simulink model "tvcControlModel"  (R2017a)
settings: Solver=VariableStepAuto  StartTime=0.0  StopTime=inf  MaxStep=0.01  RelTol=1e-3
values from neighbouring files (symbols this model uses):
  A = 0.5    [script.m]
  Cd = 1.75    [script.m]
  g = 9.81    [script.m]
  m = 0.5    [script.m]
  r = 0.28    [script.m]
  rA = 1.229    [script.m]
  Th = 11.2    [script.m]
  time = 5    [script.m]
undefined symbols (not defined in the file or in its folder): sigbuilder_block
libraries: simulink_extras x7, simulink x7, shared3dof x1, aerolibanim x1
settings Model: Creator=Jafar Iqbal  LastModifiedBy=Jafar Iqbal
settings SolverCC: AlgebraicLoopSolver=LineSearch
settings HardwareCC: TargetBitPerPointer=64  TargetBitPerSizeT=64  TargetBitPerPtrDiffT=64  TargetLongLongMode=on  TargetIntDivRoundTo=Zero  TargetEndianess=LittleEndian  TargetWordSize=64  TargetHWDeviceType=MATLAB Host  ProdEqTarget=off
settings RTWCC: SystemTargetFile=rsim.tlc  TemplateMakefile=rsim_default_tmf  Description=Rapid Simulation Target  TargetLang=C++
settings RSimTargetCC: TargetLangStandard=C++03 (ISO)  GeneratePreprocessorConditionals=Use local settings

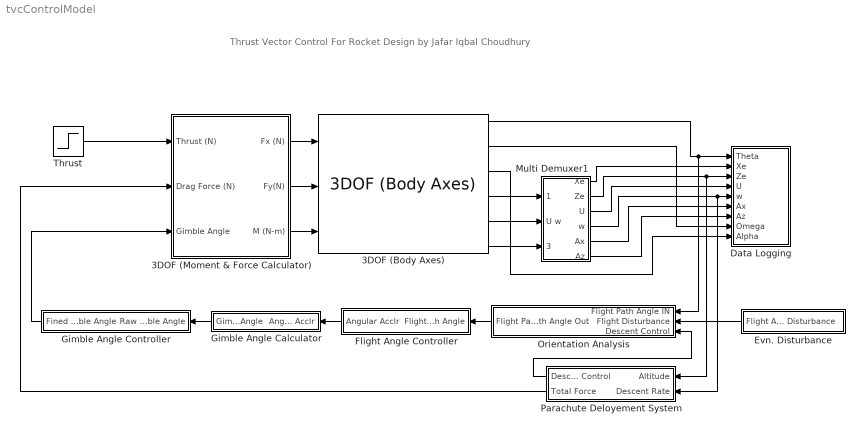
== system tvcControlModel ==
  note: Thrust Vector Control For Rocket
      | Design by Jafar Iqbal Choudhury
  3DOF (Body Axes) : shared3dof/3DOF (Body Axes)  units=Metric (MKS)  mtype=Fixed  v_ini=0  theta_ini=0  alpha_ini=0  q_ini=0  pos_ini=[0 0]  mass=m  mass_e=0.5  mass_f=3.0  Iyy=In  Iyy_e=0.5  Iyy_f=3.0  g_in=Internal  g=-9.81  vre_flag=on  abi_flag=off
  3DOF (Moment & Force Calculator) : Subsystem
  Data Logging : Subsystem
  Evn. Disturbance : Subsystem
  Flight Angle Controller : Subsystem
  Gimble Angle Calculator : Subsystem
  Gimble Angle Controller : Subsystem
  Multi Demuxer1 : Subsystem
  Orientation Analysis : Subsystem
  Parachute Deloyement System : Subsystem
  Thrust : Step  Time=time  Before=Th  After=0  SampleTime=0
  wires:
  3DOF (Moment & Force Calculator)/3(M (N-m)) -> 3DOF (Body Axes)/3
  3DOF (Moment & Force Calculator)/2(Fy(N)) -> 3DOF (Body Axes)/2
  3DOF (Moment & Force Calculator)/1(Fx (N)) -> 3DOF (Body Axes)/1
  Thrust/1 -> 3DOF (Moment & Force Calculator)/1(Thrust (N))
  3DOF (Body Axes)/4 -> Multi Demuxer1/1(Xe-Ze)
  3DOF (Body Axes)/5 -> Multi Demuxer1/2(U w)
  3DOF (Body Axes)/6 -> Multi Demuxer1/3(Ax - Az)
  Gimble Angle Controller/1(Fined Gimble Angle) -> 3DOF (Moment & Force Calculator)/3(Gimble Angle)
  Multi Demuxer1/2(Ze) -> Data Logging/3(Ze), Parachute Deloyement System/1(Altitude)
  3DOF (Body Axes)/1 -> Orientation Analysis/1(Flight Path Angle IN), Data Logging/1(Theta)
  Multi Demuxer1/1(Xe) -> Data Logging/2(Xe)
  Multi Demuxer1/3(U) -> Data Logging/4(U)
  Multi Demuxer1/5(Ax) -> Data Logging/6(Ax)
  Multi Demuxer1/6(Az) -> Data Logging/7(Az)
  3DOF (Body Axes)/2 -> Data Logging/8(Omega)
  3DOF (Body Axes)/3 -> Data Logging/9(Alpha)
  Multi Demuxer1/4(w) -> Parachute Deloyement System/2(Descent Rate), Data Logging/5(w)
  Evn. Disturbance/1(Flight Angle Disturbance) -> Orientation Analysis/2(Flight Disturbance)
  Gimble Angle Calculator/1(Gimble Angle) -> Gimble Angle Controller/1(Raw Gimble Angle)
  Flight Angle Controller/1(Angular Acclr) -> Gimble Angle Calculator/1(Angular Acclr)
  Orientation Analysis/1(Flight Path Angle Out) -> Flight Angle Controller/1(Flight Path Angle)
  Parachute Deloyement System/2(Total Force) -> 3DOF (Moment & Force Calculator)/2(Drag Force (N))
  Parachute Deloyement System/1(Descent Control) -> Orientation Analysis/3(Descent Control)

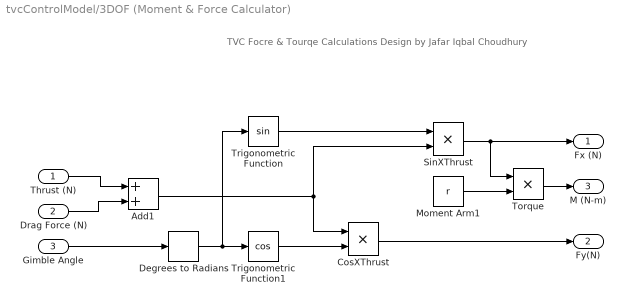
== system tvcControlModel/3DOF (Moment & Force Calculator) ==
  note: TVC Focre & Tourqe Calculations
      | Design by Jafar Iqbal Choudhury
  Thrust (N) : Inport
  Drag Force (N) : Inport  Port=2
  Gimble Angle : Inport  Port=3
  Add1 : Sum
  CosXThrust : Product
  Degrees to Radians : simulink_extras/Transformations/Degrees to Radians
  Moment Arm1 : Constant  Value=r
  SinXThrust : Product
  Torque : Product
  Trigonometric Function : Trigonometry
  Trigonometric Function1 : Trigonometry  Operator=cos
  Fx (N) : Outport
  Fy(N) : Outport  Port=2
  M (N-m) : Outport  Port=3
  wires:
  Degrees to Radians/1 -> Trigonometric Function/1, Trigonometric Function1/1
  SinXThrust/1 -> Torque/1, Fx (N)/1
  Trigonometric Function/1 -> SinXThrust/1
  Torque/1 -> M (N-m)/1
  Gimble Angle/1 -> Degrees to Radians/1
  Moment Arm1/1 -> Torque/2
  Trigonometric Function1/1 -> CosXThrust/2
  Thrust (N)/1 -> Add1/1
  Drag Force (N)/1 -> Add1/2
  Add1/1 -> SinXThrust/2, CosXThrust/1
  CosXThrust/1 -> Fy(N)/1

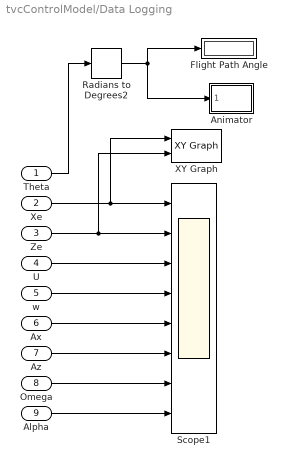
== system tvcControlModel/Data Logging ==
  Theta : Inport
  Xe : Inport  Port=2
  Ze : Inport  Port=3
  U : Inport  Port=4
  w : Inport  Port=5
  Ax : Inport  Port=6
  Az : Inport  Port=7
  Omega : Inport  Port=8
  Alpha : Inport  Port=9
  Animator : Subsystem
  Flight Path Angle : Display
  Radians to Degrees2 : simulink_extras/Transformations/Radians to Degrees
  Scope1 : Scope  NumInputPorts=8
  XY Graph : simulink/Sinks/XY Graph  xmin=-250  xmax=250  ymin=0  ymax=400  st=-1
  wires:
  Radians to Degrees2/1 -> Animator/1(FPA Input), Flight Path Angle/1
  Theta/1 -> Radians to Degrees2/1
  Ax/1 -> Scope1/5
  Az/1 -> Scope1/6
  Ze/1 -> XY Graph/2, Scope1/2
  Xe/1 -> XY Graph/1, Scope1/1
  Omega/1 -> Scope1/7
  Alpha/1 -> Scope1/8
  U/1 -> Scope1/3
  w/1 -> Scope1/4

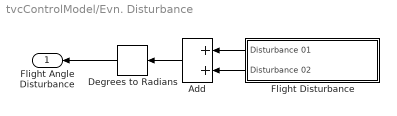
== system tvcControlModel/Evn. Disturbance ==
  Add : Sum
  Degrees to Radians : simulink_extras/Transformations/Degrees to Radians
  Flight Disturbance : Subsystem  Tag=STV Subsys  LoadFcn=sigbuilder_block('load');  StartFcn=sigbuilder_block('start');  StopFcn=sigbuilder_block('stop');  ClipboardFcn=sigbuilder_block('clipboard');  mask(Sigbuilder block){tuvar=[0:10]}
      mask help: Simulink:masks:SigbuilderBlock_MD
      mask init:
      | if ~strcmp(get_param(bdroot(gcbh),'SimulationStatus'),'stopped') tuvar = sigbuilder_block('maskInit'); end
      settings: CopyFcn=sigbuilder_block('copy');  DeleteFcn=sigbuilder_block('delete');  ModelCloseFcn=sigbuilder_block('modelClose');  PreSaveFcn=sigbuilder_block('preSave');  PauseFcn=sigbuilder_block('pause');  ContinueFcn=sigbuilder_block('continue');  NameChangeFcn=sigbuilder_block('namechange');  OpenFcn=sigbuilder_block('open',[309.75 207 550.5 483 ]);  CloseFcn=sigbuilder_block('close');
      mask Display: plot(0, 0, 100, 100,[2, 2, 32, 32, 2], [68, 8, 8, 68, 68],[32, 2], [38, 38], [32, 19, 2],[53, 60, 44], [32, 17, 17, 2],[16, 16, 31, 31]);txt = getActiveGroup(gcbh);text(2, 100, txt,'verticalAlignment', 'top');
  Flight Angle Disturbance : Outport
  wires:
  Degrees to Radians/1 -> Flight Angle Disturbance/1
  Flight Disturbance/1(Disturbance 01) -> Add/1
  Add/1 -> Degrees to Radians/1
  Flight Disturbance/2(Disturbance 02) -> Add/2

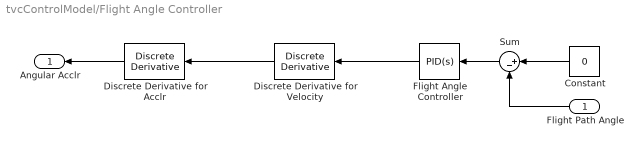
== system tvcControlModel/Flight Angle Controller ==
  Flight Path Angle : Inport
  Constant : Constant  Value=0
  Discrete Derivative for Acclr : simulink/Discrete/Discrete Derivative  gainval=1  ICPrevScaledInput=0.0  OutMin=[]  OutMax=[]  OutDataType=fixdt(1, 16)  OutScaling=2^-10  DoSatur=off
  Discrete Derivative for Velocity : simulink/Discrete/Discrete Derivative  gainval=0.5  ICPrevScaledInput=0.0  OutMin=[]  OutMax=[]  OutDataType=fixdt(1, 16)  OutScaling=2^-10  DoSatur=off
  Flight Angle Controller : simulink/Continuous/PID Controller  Controller=PID  TimeDomain=Continuous-time  SampleTime=-1  IntegratorMethod=Forward Euler  FilterMethod=Forward Euler  Form=Parallel  UseFilter=on  ControllerParametersSource=internal  P=0.179799982989109  I=4.81446374346561  D=-0.0354522581673334  N=5.07160875734514  InitialConditionSource=internal  InitialConditionForIntegrator=0  InitialConditionForFilter=0  ExternalReset=none  LimitOutput=off  UpperSaturationLimit=inf  LowerSaturationLimit=-inf  LinearizeAsGain=on  AntiWindupMode=none  Kb=1  TrackingMode=off  Kt=1  PParamMin=[]  PParamMax=[]  IParamMin=[]  IParamMax=[]  DParamMin=[]  DParamMax=[]  NParamMin=[]  NParamMax=[]  KbParamMin=[]  KbParamMax=[]  KtParamMin=[]  KtParamMax=[]  POutMin=[]  POutMax=[]  IOutMin=[]  IOutMax=[]  DOutMin=[]  DOutMax=[]  NOutMin=[]  NOutMax=[]  KbOutMin=[]  KbOutMax=[]  KtOutMin=[]  KtOutMax=[]  IntegratorOutMin=[]  IntegratorOutMax=[]  FilterOutMin=[]  FilterOutMax=[]  SumOutMin=[]  SumOutMax=[]  SumI1OutMin=[]  SumI1OutMax=[]  SumI2OutMin=[]  SumI2OutMax=[]  SumI3OutMin=[]  SumI3OutMax=[]  SumDOutMin=[]  SumDOutMax=[]  SaturationOutMin=[]  SaturationOutMax=[]  IntegratorContinuousStateAttributes=''  IntegratorStateMustResolveToSignalObject=off  IntegratorRTWStateStorageClass=Auto  FilterContinuousStateAttributes=''  FilterStateMustResolveToSignalObject=off  FilterRTWStateStorageClass=Auto  DifferentiatorICPrevScaledInput=0  DifferentiatorOutMin=[]  DifferentiatorOutMax=[]  InitialConditionSetting=State (most efficient)
  Sum : Sum  Inputs=|+-
  Angular Acclr : Outport
  wires:
  Discrete Derivative for Acclr/1 -> Angular Acclr/1
  Discrete Derivative for Velocity/1 -> Discrete Derivative for Acclr/1
  Flight Path Angle/1 -> Sum/2
  Sum/1 -> Flight Angle Controller/1
  Constant/1 -> Sum/1
  Flight Angle Controller/1 -> Discrete Derivative for Velocity/1

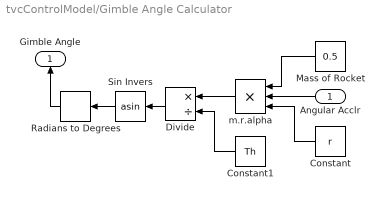
== system tvcControlModel/Gimble Angle Calculator ==
  Angular Acclr : Inport
  Constant : Constant  Value=r
  Constant1 : Constant  Value=Th
  Divide : Product  Inputs=*/
  Mass of Rocket : Constant  Value=0.5
  Radians to Degrees : simulink_extras/Transformations/Radians to Degrees
  Sin Invers : Trigonometry  Operator=asin
  m.r.alpha : Product  Inputs=3
  Gimble Angle : Outport
  wires:
  Constant/1 -> m.r.alpha/3
  Angular Acclr/1 -> m.r.alpha/2
  Divide/1 -> Sin Invers/1
  Sin Invers/1 -> Radians to Degrees/1
  Mass of Rocket/1 -> m.r.alpha/1
  m.r.alpha/1 -> Divide/1
  Radians to Degrees/1 -> Gimble Angle/1
  Constant1/1 -> Divide/2

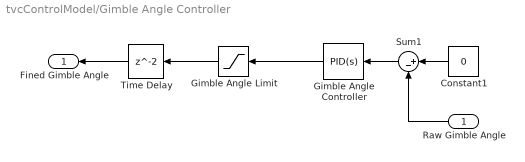
== system tvcControlModel/Gimble Angle Controller ==
  Raw Gimble Angle : Inport
  Constant1 : Constant  Value=0
  Gimble Angle Controller : simulink/Continuous/PID Controller  Controller=PID  TimeDomain=Continuous-time  SampleTime=-1  IntegratorMethod=Forward Euler  FilterMethod=Forward Euler  Form=Parallel  UseFilter=on  ControllerParametersSource=internal  P=-1.1585785296482  I=-0.462318901837309  D=-0.0612378009118757  N=3.02027555618535  InitialConditionSource=internal  InitialConditionForIntegrator=0  InitialConditionForFilter=0  ExternalReset=none  LimitOutput=off  UpperSaturationLimit=inf  LowerSaturationLimit=-inf  LinearizeAsGain=on  AntiWindupMode=none  Kb=1  TrackingMode=off  Kt=1  PParamMin=[]  PParamMax=[]  IParamMin=[]  IParamMax=[]  DParamMin=[]  DParamMax=[]  NParamMin=[]  NParamMax=[]  KbParamMin=[]  KbParamMax=[]  KtParamMin=[]  KtParamMax=[]  POutMin=[]  POutMax=[]  IOutMin=[]  IOutMax=[]  DOutMin=[]  DOutMax=[]  NOutMin=[]  NOutMax=[]  KbOutMin=[]  KbOutMax=[]  KtOutMin=[]  KtOutMax=[]  IntegratorOutMin=[]  IntegratorOutMax=[]  FilterOutMin=[]  FilterOutMax=[]  SumOutMin=[]  SumOutMax=[]  SumI1OutMin=[]  SumI1OutMax=[]  SumI2OutMin=[]  SumI2OutMax=[]  SumI3OutMin=[]  SumI3OutMax=[]  SumDOutMin=[]  SumDOutMax=[]  SaturationOutMin=[]  SaturationOutMax=[]  IntegratorContinuousStateAttributes=''  IntegratorStateMustResolveToSignalObject=off  IntegratorRTWStateStorageClass=Auto  FilterContinuousStateAttributes=''  FilterStateMustResolveToSignalObject=off  FilterRTWStateStorageClass=Auto  DifferentiatorICPrevScaledInput=0  DifferentiatorOutMin=[]  DifferentiatorOutMax=[]  InitialConditionSetting=State (most efficient)
  Gimble Angle Limit : Saturate  UpperLimit=5  LowerLimit=-5
  Sum1 : Sum  Inputs=|+-
  Time Delay : Delay
  Fined Gimble Angle : Outport
  wires:
  Sum1/1 -> Gimble Angle Controller/1
  Constant1/1 -> Sum1/1
  Raw Gimble Angle/1 -> Sum1/2
  Gimble Angle Limit/1 -> Time Delay/1
  Time Delay/1 -> Fined Gimble Angle/1
  Gimble Angle Controller/1 -> Gimble Angle Limit/1

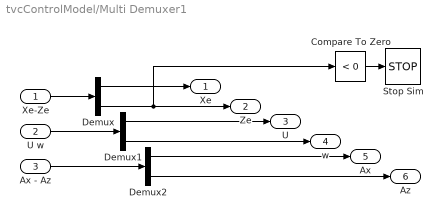
== system tvcControlModel/Multi Demuxer1 ==
  Xe-Ze : Inport
  U w : Inport  Port=2
  Ax - Az : Inport  Port=3
  Compare To Zero : simulink/Logic and Bit Operations/Compare To Zero  relop=<  OutDataTypeStr=boolean
  Demux : Demux  Outputs=2
  Demux1 : Demux  Outputs=2
  Demux2 : Demux  Outputs=2
  Stop Sim : Stop
  Xe : Outport
  Ze : Outport  Port=2
  U : Outport  Port=3
  w : Outport  Port=4
  Ax : Outport  Port=5
  Az : Outport  Port=6
  wires:
  Compare To Zero/1 -> Stop Sim/1
  Demux1/1 -> U/1
  Demux/2 -> Ze/1, Compare To Zero/1
  Demux2/1 -> Ax/1
  Xe-Ze/1 -> Demux/1
  Demux2/2 -> Az/1
  Demux1/2 -> w/1
  Demux/1 -> Xe/1
  U w/1 -> Demux1/1
  Ax - Az/1 -> Demux2/1

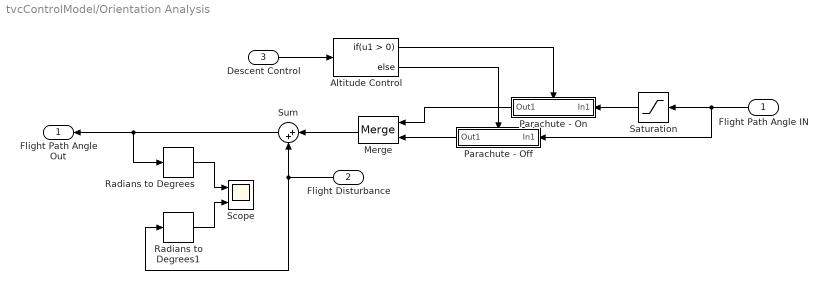
== system tvcControlModel/Orientation Analysis ==
  Flight Path Angle IN : Inport
  Flight Disturbance : Inport  Port=2
  Descent Control : Inport  Port=3
  Altitude Control : If
  Merge : Merge
  Parachute - Off : Subsystem  TreatAsAtomicUnit=on
  Parachute - On : Subsystem  TreatAsAtomicUnit=on
  Radians to Degrees : simulink_extras/Transformations/Radians to Degrees
  Radians to Degrees1 : simulink_extras/Transformations/Radians to Degrees
  Saturation : Saturate  UpperLimit=3  LowerLimit=-3
  Scope : Scope  NumInputPorts=2
  Sum : Sum  Inputs=|++
  Flight Path Angle Out : Outport
  wires:
  Radians to Degrees/1 -> Scope/1
  Flight Disturbance/1 -> Radians to Degrees1/1, Sum/2
  Sum/1 -> Flight Path Angle Out/1, Radians to Degrees/1
  Radians to Degrees1/1 -> Scope/2
  Altitude Control/1 -> Parachute - On/Action
  Altitude Control/2 -> Parachute - Off/Action
  Parachute - Off/1(Out1) -> Merge/2
  Parachute - On/1(Out1) -> Merge/1
  Merge/1 -> Sum/1
  Descent Control/1 -> Altitude Control/1
  Saturation/1 -> Parachute - On/1(In1)
  Flight Path Angle IN/1 -> Parachute - Off/1(In1), Saturation/1

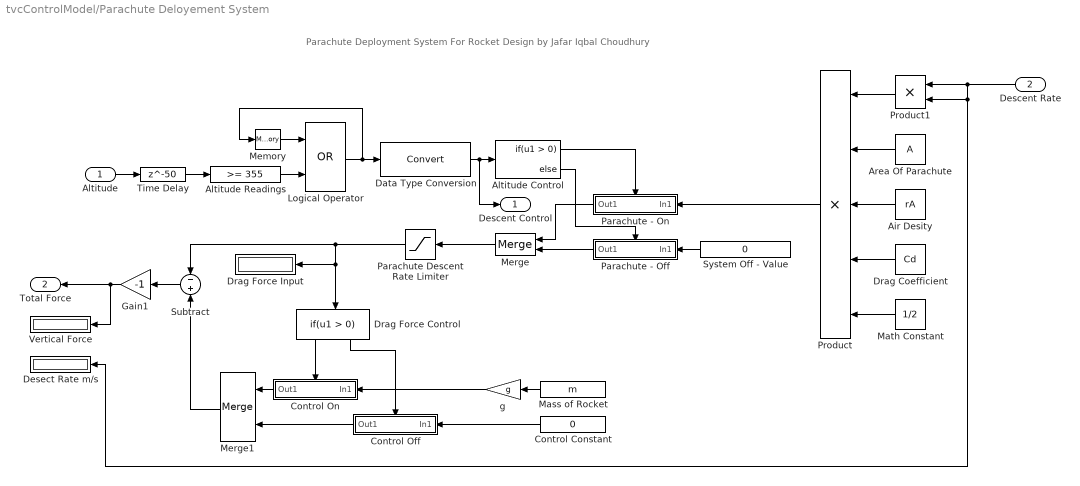
== system tvcControlModel/Parachute Deloyement System ==
  note: Parachute Deployment System For Rocket
      | Design by Jafar Iqbal Choudhury
  Altitude : Inport
  Descent Rate : Inport  Port=2
  Air Desity : Constant  Value=rA
  Altitude Control : If
  Altitude Readings : simulink/Logic and Bit Operations/Compare To Constant  relop=>=  const=355  OutDataTypeStr=boolean
  Area Of Parachute : Constant  Value=A
  Control Constant : Constant  Value=0
  Control Off : Subsystem  TreatAsAtomicUnit=on
  Control On : Subsystem  TreatAsAtomicUnit=on
  Data Type Conversion : DataTypeConversion
  Desect Rate m/s : Display
  Drag Coefficient : Constant  Value=Cd
  Drag Force Control : If
  Drag Force Input : Display
  Gain1 : Gain  Gain=-1
  Logical Operator : Logic  Operator=OR  AllPortsSameDT=off
  Mass of Rocket : Constant  Value=m
  Math Constant : Constant  Value=1/2
  Memory : Memory  InheritSampleTime=on
  Merge : Merge
  Merge1 : Merge
  Parachute - Off : Subsystem  TreatAsAtomicUnit=on
  Parachute - On : Subsystem  TreatAsAtomicUnit=on
  Parachute Descent Rate Limiter : Saturate  UpperLimit=15  LowerLimit=-15
  Product : Product  Inputs=5
  Product1 : Product
  Subtract : Sum  Inputs=-+
  System Off - Value : Constant  Value=0
  Time Delay : Delay  DelayLength=50
  Vertical Force : Display
  g : Gain  Gain=g
  Descent Control : Outport
  Total Force : Outport  Port=2
  wires:
  Parachute - Off/1(Out1) -> Merge/2
  Altitude Control/2 -> Parachute - Off/Action
  Parachute - On/1(Out1) -> Merge/1
  Altitude Control/1 -> Parachute - On/Action
  Product/1 -> Parachute - On/1(In1)
  System Off - Value/1 -> Parachute - Off/1(In1)
  Merge/1 -> Parachute Descent Rate Limiter/1
  Memory/1 -> Logical Operator/1
  Altitude Readings/1 -> Logical Operator/2
  Altitude/1 -> Time Delay/1
  Time Delay/1 -> Altitude Readings/1
  Logical Operator/1 -> Data Type Conversion/1, Memory/1
  Data Type Conversion/1 -> Descent Control/1, Altitude Control/1
  Mass of Rocket/1 -> g/1
  Subtract/1 -> Gain1/1
  Merge1/1 -> Subtract/2
  Control Off/1(Out1) -> Merge1/2
  Control On/1(Out1) -> Merge1/1
  g/1 -> Control On/1(In1)
  Drag Force Control/1 -> Control On/Action
  Drag Force Control/2 -> Control Off/Action
  Control Constant/1 -> Control Off/1(In1)
  Gain1/1 -> Total Force/1, Vertical Force/1
  Product1/1 -> Product/1
  Drag Coefficient/1 -> Product/4
  Air Desity/1 -> Product/3
  Area Of Parachute/1 -> Product/2
  Descent Rate/1 -> Desect Rate m/s/1, Product1/2, Product1/1
  Math Constant/1 -> Product/5
  Parachute Descent Rate Limiter/1 -> Subtract/1, Drag Force Control/1, Drag Force Input/1

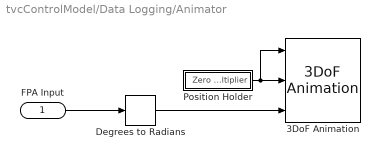
== system tvcControlModel/Data Logging/Animator ==
  FPA Input : Inport
  3DoF Animation : aerolibanim/3DoF Animation  u1=[-30 30 -30 30 -30 30]  u2=0.05  u3=1  u5=Fly alongside  u6=[0 50 0]  u7=45  u8=on
      settings: SourceProductName=Aerospace Blockset  SourceProductBaseCode=AE
  Degrees to Radians : simulink_extras/Transformations/Degrees to Radians
  Position Holder : Subsystem
  wires:
  FPA Input/1 -> Degrees to Radians/1
  Position Holder/1(Zero Multiplier) -> 3DoF Animation/1, 3DoF Animation/2
  Degrees to Radians/1 -> 3DoF Animation/3

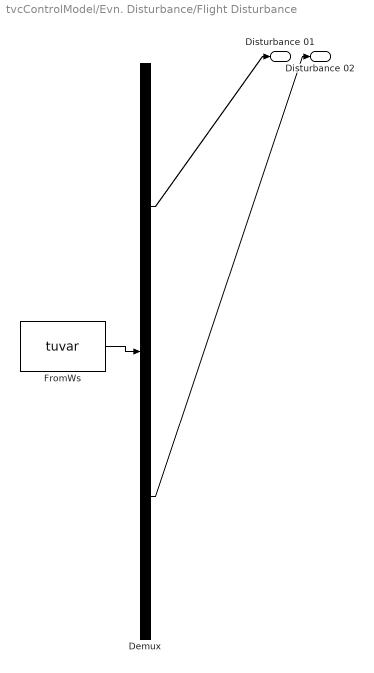
== system tvcControlModel/Evn. Disturbance/Flight Disturbance ==
  Demux : Demux  Tag=STV Demux  Outputs=2
  FromWs : FromWorkspace  Tag=STV FromWs  VariableName=tuvar  SampleTime=0
      SigBuilderData=|
      | common.afterFinalStr = 'Extrapolate'
      | common.sampleTime = 0
      | dataSet.timeRange = [0 10]
      | dataSet.name = 'Env Disturbance'
      | sbobj.Groups.Name = 'Env Disturbance'
      | sbobj.Groups.Signals(1).Name = 'Disturbance 01'
      | sbobj.Groups.Signals(1).XData = [0 1 1 2 2 10]
      | sbobj.Groups.Signals(1).YData = [0 0 5 5 0 0]
      | sbobj.Groups.Signals(2).Name = 'Disturbance 02'
      | sbobj.Groups.Signals(2).XData = [0 3 3 4 4 10]
      | sbobj.Groups.Signals(2).YData = [0 0 -5 -5 0 0]
  Disturbance 01 : Outport  Tag=STV Outport
  Disturbance 02 : Outport  Tag=STV Outport  Port=2
  wires:
  FromWs/1 -> Demux/1
  Demux/1 -> Disturbance 01/1
  Demux/2 -> Disturbance 02/1

== system tvcControlModel/Orientation Analysis/Parachute - Off ==
  In1 : Inport
  Action Port : ActionPort  ActionType=else
  Out1 : Outport
  wires:
  In1/1 -> Out1/1

== system tvcControlModel/Orientation Analysis/Parachute - On ==
  In1 : Inport
  Action Port : ActionPort  ActionType=then
  Out1 : Outport
  wires:
  In1/1 -> Out1/1

== system tvcControlModel/Parachute Deloyement System/Control Off ==
  In1 : Inport
  Action Port : ActionPort  ActionType=else
  Out1 : Outport
  wires:
  In1/1 -> Out1/1

== system tvcControlModel/Parachute Deloyement System/Control On ==
  In1 : Inport
  Action Port : ActionPort  ActionType=then
  Out1 : Outport
  wires:
  In1/1 -> Out1/1

== system tvcControlModel/Parachute Deloyement System/Parachute - Off ==
  In1 : Inport
  Action Port : ActionPort  ActionType=else
  Out1 : Outport
  wires:
  In1/1 -> Out1/1

== system tvcControlModel/Parachute Deloyement System/Parachute - On ==
  In1 : Inport
  Action Port : ActionPort  ActionType=then
  Out1 : Outport
  wires:
  In1/1 -> Out1/1

== system tvcControlModel/Data Logging/Animator/Position Holder ==
  Constant : Constant
  Constant1 : Constant
  Mux : Mux  Inputs=2
  Zero Multiplier : Outport
  wires:
  Constant1/1 -> Mux/2
  Mux/1 -> Zero Multiplier/1
  Constant/1 -> Mux/1
